simulink model "trig"  (Simulink 6.6)
settings: Solver=FixedStepDiscrete  StartTime=0.0  StopTime=10.0  FixedStep=1  RelTol=1e-3
settings Model: Creator=ksmyth  LastModifiedBy=hnine

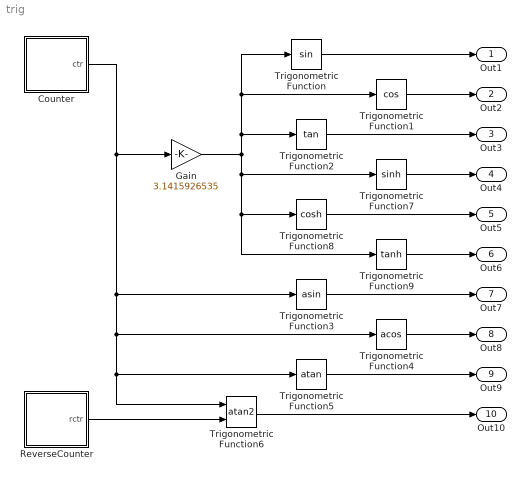
== system trig ==
  Counter : Stateflow chart
  Gain : Gain  Gain=3.1415926535
  ReverseCounter : Stateflow chart
  Trigonometric Function : Trigonometry
  Trigonometric Function1 : Trigonometry  Operator=cos
  Trigonometric Function2 : Trigonometry  Operator=tan
  Trigonometric Function3 : Trigonometry  Operator=asin
  Trigonometric Function4 : Trigonometry  Operator=acos
  Trigonometric Function5 : Trigonometry  Operator=atan
  Trigonometric Function6 : Trigonometry  Operator=atan2
  Trigonometric Function7 : Trigonometry  Operator=sinh
  Trigonometric Function8 : Trigonometry  Operator=cosh
  Trigonometric Function9 : Trigonometry  Operator=tanh
  Out1 : Outport
  Out2 : Outport  Port=2
  Out3 : Outport  Port=3
  Out4 : Outport  Port=4
  Out5 : Outport  Port=5
  Out6 : Outport  Port=6
  Out7 : Outport  Port=7
  Out8 : Outport  Port=8
  Out9 : Outport  Port=9
  Out10 : Outport  Port=10
  wires:
  Counter/1(ctr) -> Trigonometric Function3/1, Trigonometric Function5/1, Trigonometric Function6/1, Trigonometric Function4/1, Gain/1
  Trigonometric Function/1 -> Out1/1
  Trigonometric Function1/1 -> Out2/1
  Trigonometric Function2/1 -> Out3/1
  Trigonometric Function3/1 -> Out7/1
  Trigonometric Function4/1 -> Out8/1
  Trigonometric Function5/1 -> Out9/1
  Trigonometric Function6/1 -> Out10/1
  Trigonometric Function7/1 -> Out4/1
  Trigonometric Function8/1 -> Out5/1
  Trigonometric Function9/1 -> Out6/1
  ReverseCounter/1(rctr) -> Trigonometric Function6/2
  Gain/1 -> Trigonometric Function/1, Trigonometric Function1/1, Trigonometric Function2/1, Trigonometric Function7/1, Trigonometric Function8/1, Trigonometric Function9/1

== stateflow chart Counter ==
  state s1
  (default) -> s1
  s1 -> s1 [order 1] : [ctr <1 ] / ctr = ctr+0.2;
  s1 -> s1 [order 2] : [ctr >= 1] / ctr = -0.8;
  data: ctr output double =1

== stateflow chart ReverseCounter ==
  state s1
  note: 2*pi
  (default) -> s1
  s1 -> s1 [order 1] : [rctr >-6.2831853 ] / rctr = rctr-0.02;
  s1 -> s1 [order 2] : [rctr <= -6.2831853] / rctr = 6.2831853;
  data: rctr output double =1
